simulink model "metronomo"  (Simulink 8.1)
settings: Solver=ode45  StartTime=0.0  StopTime=10.0  RelTol=1e-6
undefined symbols (not defined in the file): beta, g, J, k, L, l, M, m, x0
settings Model: Creator=g  LastModifiedBy=Diogo Bras

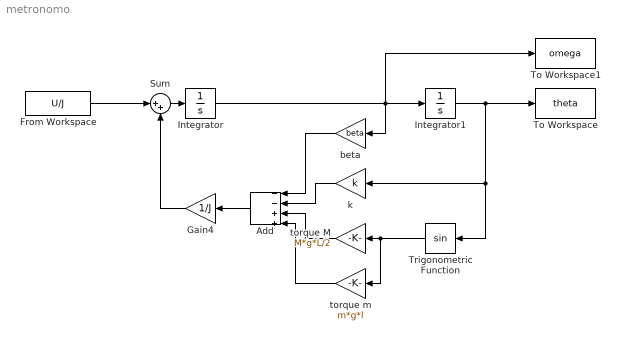
== system metronomo ==
  Add : Sum  Inputs=--++
  From Workspace : FromWorkspace  VariableName=U/J  SampleTime=0
  Gain4 : Gain  Gain=1/J
  Integrator : Integrator  InitialCondition=x0(2)
  Integrator1 : Integrator  InitialCondition=x0(1)
  Sum : Sum  Inputs=|++
  To Workspace : ToWorkspace  VariableName=theta  SampleTime=-1
  To Workspace1 : ToWorkspace  VariableName=omega  SampleTime=-1
  Trigonometric Function : Trigonometry
  beta : Gain  Gain=beta
  k : Gain  Gain=k
  torque M : Gain  Gain=M*g*L/2
  torque m : Gain  Gain=m*g*l
  wires:
  Integrator/1 -> Integrator1/1, beta/1, To Workspace1/1
  Trigonometric Function/1 -> torque M/1, torque m/1
  Integrator1/1 -> Trigonometric Function/1, k/1, To Workspace/1
  beta/1 -> Add/1
  k/1 -> Add/2
  torque M/1 -> Add/3
  torque m/1 -> Add/4
  Add/1 -> Gain4/1
  Gain4/1 -> Sum/2
  Sum/1 -> Integrator/1
  From Workspace/1 -> Sum/1
